simulink model "SecRwLtStBkReclnCtrl"  (R2024b)
settings: Solver=FixedStepDiscrete  StartTime=0.0  StopTime=10.0  FixedStep=0.01  RelTol=1e-3
undefined symbols (not defined in the file or in its folder): KeSMSuMdMotFinshdTm_Val, KeSMSuMdRetryTm1_Val, KeSMSuModeReqDurgTm_Val, KeSMSwSecRwLtStBkReclnEnTrigBitMask_Val
libraries: StCtrlLibBkRecln x1
settings Model: ModifiedHistory=2025.12.04 MD10增加防夹后退出机制  Creator=sn2xws  LastModifiedBy=sn55gm
settings SolverCC: AlgebraicLoopSolver=TrustRegion
settings DataIOCC: SaveFormat=StructureWithTime  ReturnWorkspaceOutputs=off
settings OptimizationCC: DefaultParameterBehavior=Inlined  EnhancedBackFolding=on  PassReuseOutputArgsAs=Individual arguments  ZeroExternalMemoryAtStartup=off  ZeroInternalMemoryAtStartup=off  OptimizeBlockOrder=speed  DifferentSizesBufferReuse=on  OptimizationCustomize=off  EfficientTunableParamExpr=on
settings DebuggingCC: ParameterTunabilityLossMsg=error  UnconnectedInputMsg=warning  UnconnectedOutputMsg=warning  UnconnectedLineMsg=warning  ArithmeticOperatorsInVariantConditions=warning
settings ModelReferenceCC: EnableRefExpFcnMdlSchedulingChecks=on  ModelReferenceNumInstancesAllowed=Single
settings SFSimCC: MATLABDynamicMemAlloc=off  CustomCodeUndefinedFunction=UseInterfaceOnly
settings RTWCC: Description=AUTOSAR  SystemTargetFile=autosar.tlc  GenCodeOnly=on  TemplateMakefile=ert_default_tmf  GenerateReport=on  IncludeHyperlinkInReport=on  LaunchReport=on  DataTypeReplacement=CDataTypesFixedWidth  GenerateTraceInfo=on  GenerateTraceReport=on  GenerateTraceReportSl=on  GenerateTraceReportSf=on  GenerateTraceReportEml=on  GenerateCodeMetricsReport=on  GPUComputeCapability=3.5
settings CodeAppCC: ForceParamTrailComments=on  IgnoreCustomStorageClasses=off  OperatorAnnotations=on  SimulinkDataObjDesc=on  SFDataObjDesc=on  InsertBlockDesc=on
settings STFCustomTargetCC: TargetLangStandard=C99 (ISO)  MultiwordLength=256  ParMdlRefBuildCompliant=on  CompOptLevelCompliant=on  IncludeMdlTerminateFcn=off  CombineOutputUpdateFcns=on  SuppressErrorStatus=on  ERTCustomFileBanners=on  SupportNonFinite=off  SupportComplex=off  SupportContinuousTime=off  SupportNonInlinedSFcns=off  RemoveResetFunc=on  MATLABClassNameForMDSCustomization=Simulink.SoftwareTarget.ERTCustomization  AutosarCompliant=on  UseToolchainInfoCompliant=on  LookupTableObjectStructAxisOrder=2,1,3,4,...  LUTObjectStructOrderEvenSpacing=Size,Table,Breakpoints  SystemTargetFile=autosar.tlc
settings ERTTargetCC: TargetLangStandard=C99 (ISO)  ConcurrentExecutionCompliant=off  IncludeMdlTerminateFcn=off  SuppressErrorStatus=on  SupportNonFinite=off  SupportComplex=off  ModelStepFunctionPrototypeControlCompliant=off  CPPClassGenCompliant=off  AutosarCompliant=on  LookupTableObjectStructAxisOrder=2,1,3,4,...  LUTObjectStructOrderEvenSpacing=Size,Table,Breakpoints  ERTCustomFileTemplate=example_file_process.tlc  ERTFilePackagingFormat=Compact  BooleanTrueId=TRUE  BooleanFalseId=FALSE  DynamicArrayContainerType=coder::array

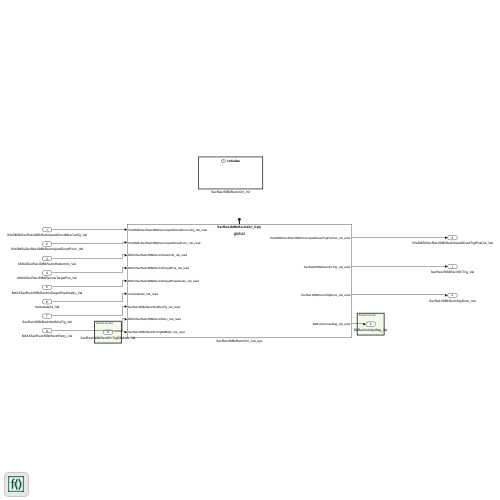
[thumbnail: Simulink's stored preview of the top-level diagram]
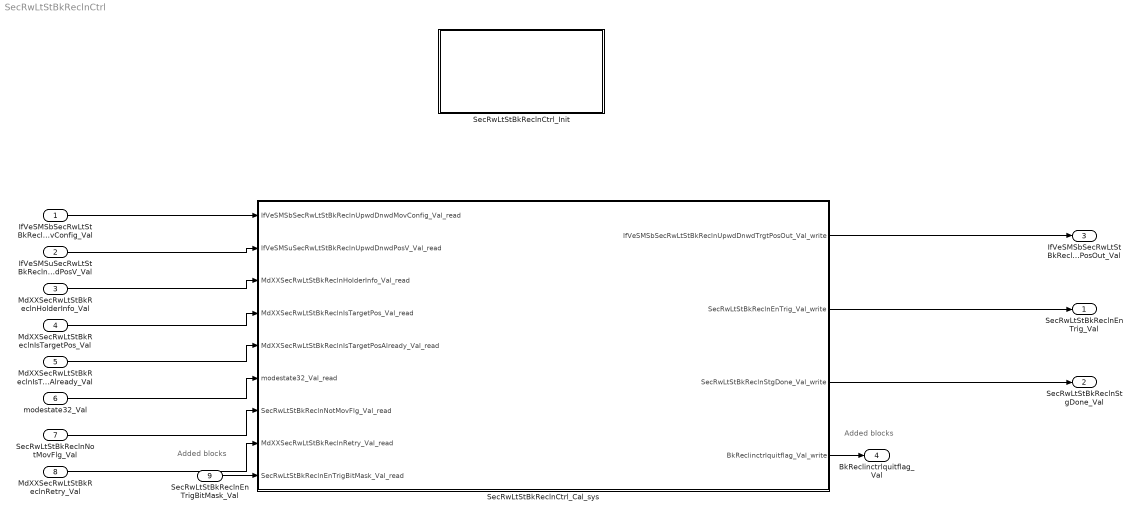
== system SecRwLtStBkReclnCtrl ==
  note: Added blocks
  note: Added blocks
  IfVeSMSbSecRwLtStBkReclnUpwdDnwdMovConfig_Val : Inport  OutDataTypeStr=boolean  PortDimensions=1
  IfVeSMSuSecRwLtStBkReclnUpwdDnwdPosV_Val : Inport  Port=2  OutDataTypeStr=boolean  PortDimensions=1
  MdXXSecRwLtStBkReclnHolderInfo_Val : Inport  Port=3  OutDataTypeStr=uint32  PortDimensions=1
  MdXXSecRwLtStBkReclnIsTargetPos_Val : Inport  Port=4  OutDataTypeStr=uint32  PortDimensions=1
  MdXXSecRwLtStBkReclnIsTargetPosAlready_Val : Inport  Port=5  OutDataTypeStr=uint32  PortDimensions=1
  modestate32_Val : Inport  Port=6  OutDataTypeStr=uint32  PortDimensions=1
  SecRwLtStBkReclnNotMovFlg_Val : Inport  Port=7  OutDataTypeStr=boolean  PortDimensions=1
  MdXXSecRwLtStBkReclnRetry_Val : Inport  Port=8  OutDataTypeStr=uint32  PortDimensions=1
  SecRwLtStBkReclnEnTrigBitMask_Val : Inport  Port=9  OutDataTypeStr=uint32  PortDimensions=1
  SecRwLtStBkReclnCtrl_Cal_sys : Subsystem
  SecRwLtStBkReclnCtrl_Init : Subsystem
  SecRwLtStBkReclnEnTrig_Val : Outport  OutDataTypeStr=boolean  PortDimensions=1  VectorParamsAs1DForOutWhenUnconnected=off
  SecRwLtStBkReclnStgDone_Val : Outport  Port=2  OutDataTypeStr=boolean  PortDimensions=1  VectorParamsAs1DForOutWhenUnconnected=off
  IfVeSMSbSecRwLtStBkReclnUpwdDnwdTrgtPosOut_Val : Outport  Port=3  OutDataTypeStr=boolean  PortDimensions=1  VectorParamsAs1DForOutWhenUnconnected=off
  BkReclinctrlquitflag_Val : Outport  Port=4  OutDataTypeStr=boolean  PortDimensions=1  VectorParamsAs1DForOutWhenUnconnected=off
  wires:
  IfVeSMSbSecRwLtStBkReclnUpwdDnwdMovConfig_Val/1 -> SecRwLtStBkReclnCtrl_Cal_sys/1(IfVeSMSbSecRwLtStBkReclnUpwdDnwdMovConfig_Val_read)
  IfVeSMSuSecRwLtStBkReclnUpwdDnwdPosV_Val/1 -> SecRwLtStBkReclnCtrl_Cal_sys/2(IfVeSMSuSecRwLtStBkReclnUpwdDnwdPosV_Val_read)
  MdXXSecRwLtStBkReclnHolderInfo_Val/1 -> SecRwLtStBkReclnCtrl_Cal_sys/3(MdXXSecRwLtStBkReclnHolderInfo_Val_read)
  MdXXSecRwLtStBkReclnIsTargetPos_Val/1 -> SecRwLtStBkReclnCtrl_Cal_sys/4(MdXXSecRwLtStBkReclnIsTargetPos_Val_read)
  MdXXSecRwLtStBkReclnIsTargetPosAlready_Val/1 -> SecRwLtStBkReclnCtrl_Cal_sys/5(MdXXSecRwLtStBkReclnIsTargetPosAlready_Val_read)
  modestate32_Val/1 -> SecRwLtStBkReclnCtrl_Cal_sys/6(modestate32_Val_read)
  SecRwLtStBkReclnNotMovFlg_Val/1 -> SecRwLtStBkReclnCtrl_Cal_sys/7(SecRwLtStBkReclnNotMovFlg_Val_read)
  SecRwLtStBkReclnCtrl_Cal_sys/1(IfVeSMSbSecRwLtStBkReclnUpwdDnwdTrgtPosOut_Val_write) -> IfVeSMSbSecRwLtStBkReclnUpwdDnwdTrgtPosOut_Val/1
  SecRwLtStBkReclnCtrl_Cal_sys/2(SecRwLtStBkReclnEnTrig_Val_write) -> SecRwLtStBkReclnEnTrig_Val/1
  SecRwLtStBkReclnCtrl_Cal_sys/3(SecRwLtStBkReclnStgDone_Val_write) -> SecRwLtStBkReclnStgDone_Val/1
  MdXXSecRwLtStBkReclnRetry_Val/1 -> SecRwLtStBkReclnCtrl_Cal_sys/8(MdXXSecRwLtStBkReclnRetry_Val_read)
  SecRwLtStBkReclnEnTrigBitMask_Val/1 -> SecRwLtStBkReclnCtrl_Cal_sys/9(SecRwLtStBkReclnEnTrigBitMask_Val_read)
  SecRwLtStBkReclnCtrl_Cal_sys/4(BkReclinctrlquitflag_Val_write) -> BkReclinctrlquitflag_Val/1

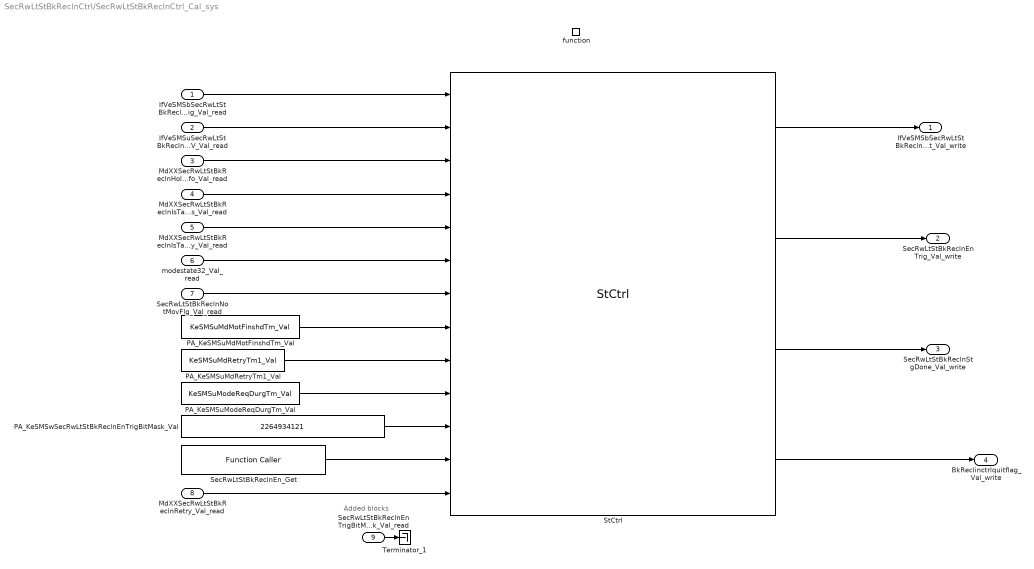
== system SecRwLtStBkReclnCtrl/SecRwLtStBkReclnCtrl_Cal_sys ==
  note: Added blocks
  IfVeSMSbSecRwLtStBkReclnUpwdDnwdMovConfig_Val_read : Inport
  IfVeSMSuSecRwLtStBkReclnUpwdDnwdPosV_Val_read : Inport  Port=2
  MdXXSecRwLtStBkReclnHolderInfo_Val_read : Inport  Port=3
  MdXXSecRwLtStBkReclnIsTargetPos_Val_read : Inport  Port=4
  MdXXSecRwLtStBkReclnIsTargetPosAlready_Val_read : Inport  Port=5
  modestate32_Val_read : Inport  Port=6
  SecRwLtStBkReclnNotMovFlg_Val_read : Inport  Port=7
  MdXXSecRwLtStBkReclnRetry_Val_read : Inport  Port=8
  SecRwLtStBkReclnEnTrigBitMask_Val_read : Inport  Port=9
  function : TriggerPort  TriggerType=function-call  IsSimulinkFunction=on  FunctionName=SecRwLtStBkReclnCtrl_Cal  VariantControl=(inherit)
  PA_KeSMSuMdMotFinshdTm_Val : Constant  Value=KeSMSuMdMotFinshdTm_Val
  PA_KeSMSuMdRetryTm1_Val : Constant  Value=KeSMSuMdRetryTm1_Val
  PA_KeSMSuModeReqDurgTm_Val : Constant  Value=KeSMSuModeReqDurgTm_Val
  PA_KeSMSwSecRwLtStBkReclnEnTrigBitMask_Val : Constant  Value=2264934121  OutDataTypeStr=uint32
  SecRwLtStBkReclnEn_Get : FunctionCaller  FunctionPrototype=data = SecRwLtStBkReclnEn_Get()  InputArgumentSpecifications=<Enter example>  OutputArgumentSpecifications=uint32(1)
  StCtrl : StCtrlLibBkRecln/StCtrl  SystemSampleTime=-1  VariantActivationTime=update diagram  AllowFlexibleInterface=on  Latency=0  AutoFrameSizeCalculation=off
  Terminator_1 : Terminator
  IfVeSMSbSecRwLtStBkReclnUpwdDnwdTrgtPosOut_Val_write : Outport  VectorParamsAs1DForOutWhenUnconnected=off
      settings: EnsureOutportIsVirtual=on
  SecRwLtStBkReclnEnTrig_Val_write : Outport  Port=2  VectorParamsAs1DForOutWhenUnconnected=off
      settings: EnsureOutportIsVirtual=on
  SecRwLtStBkReclnStgDone_Val_write : Outport  Port=3  VectorParamsAs1DForOutWhenUnconnected=off
      settings: EnsureOutportIsVirtual=on
  BkReclinctrlquitflag_Val_write : Outport  Port=4  VectorParamsAs1DForOutWhenUnconnected=off
      settings: EnsureOutportIsVirtual=on
  wires:
  StCtrl/1 -> IfVeSMSbSecRwLtStBkReclnUpwdDnwdTrgtPosOut_Val_write/1
  StCtrl/3 -> SecRwLtStBkReclnStgDone_Val_write/1
  StCtrl/2 -> SecRwLtStBkReclnEnTrig_Val_write/1
  PA_KeSMSwSecRwLtStBkReclnEnTrigBitMask_Val/1 -> StCtrl/11
  SecRwLtStBkReclnEn_Get/1 -> StCtrl/12
  PA_KeSMSuMdMotFinshdTm_Val/1 -> StCtrl/8
  PA_KeSMSuModeReqDurgTm_Val/1 -> StCtrl/10
  PA_KeSMSuMdRetryTm1_Val/1 -> StCtrl/9
  IfVeSMSbSecRwLtStBkReclnUpwdDnwdMovConfig_Val_read/1 -> StCtrl/1
  IfVeSMSuSecRwLtStBkReclnUpwdDnwdPosV_Val_read/1 -> StCtrl/2
  MdXXSecRwLtStBkReclnHolderInfo_Val_read/1 -> StCtrl/3
  MdXXSecRwLtStBkReclnIsTargetPos_Val_read/1 -> StCtrl/4
  MdXXSecRwLtStBkReclnIsTargetPosAlready_Val_read/1 -> StCtrl/5
  modestate32_Val_read/1 -> StCtrl/6
  SecRwLtStBkReclnNotMovFlg_Val_read/1 -> StCtrl/7
  MdXXSecRwLtStBkReclnRetry_Val_read/1 -> StCtrl/13
  SecRwLtStBkReclnEnTrigBitMask_Val_read/1 -> Terminator_1/1
  StCtrl/4 -> BkReclinctrlquitflag_Val_write/1

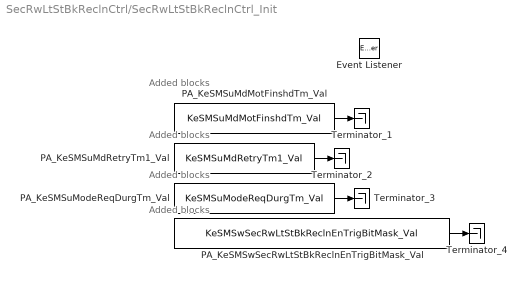
== system SecRwLtStBkReclnCtrl/SecRwLtStBkReclnCtrl_Init ==
  note: Added blocks
  note: Added blocks
  note: Added blocks
  note: Added blocks
  Event Listener : EventListener  EventName=reset
  PA_KeSMSuMdMotFinshdTm_Val : Constant  Value=KeSMSuMdMotFinshdTm_Val
  PA_KeSMSuMdRetryTm1_Val : Constant  Value=KeSMSuMdRetryTm1_Val
  PA_KeSMSuModeReqDurgTm_Val : Constant  Value=KeSMSuModeReqDurgTm_Val
  PA_KeSMSwSecRwLtStBkReclnEnTrigBitMask_Val : Constant  Value=KeSMSwSecRwLtStBkReclnEnTrigBitMask_Val
  Terminator_{1..4} (4 alike) : Terminator
  wires:
  PA_KeSMSuMdMotFinshdTm_Val/1 -> Terminator_1/1
  PA_KeSMSuMdRetryTm1_Val/1 -> Terminator_2/1
  PA_KeSMSuModeReqDurgTm_Val/1 -> Terminator_3/1
  PA_KeSMSwSecRwLtStBkReclnEnTrigBitMask_Val/1 -> Terminator_4/1
